simulink model "sus"  (Simulink 6.5)
settings: Solver=ode45  StartTime=0.0  StopTime=16  RelTol=1e-3
libraries: cdsFilt x266, cdsBitwise x92, cdsEpicsOut x84, cdsEpicsBinIn x56, cdsEpicsIn x20, cdsFiltCtrl x18, cdsMatrix x11, cdsSwitch x7, cdsWD x7, cdsFunctionCall x5, cdsRio1 x4, dac x3
(part 3 of 20)

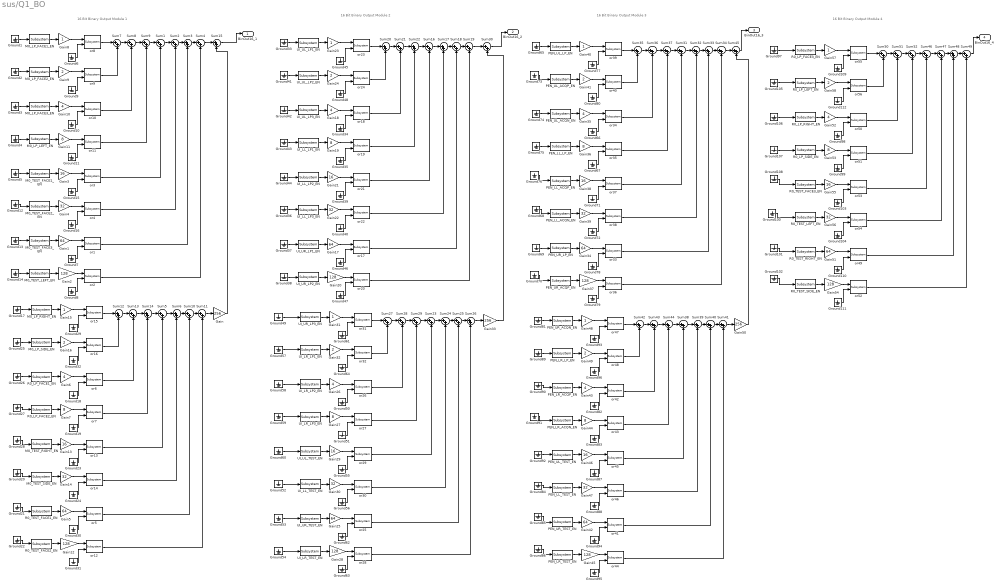
== system sus/Q1_BO ==
  note: 16 Bit Binary Output Module 1
  note: 16 Bit Binary Output Module 2
  note: 16 Bit Binary Output Module 3
  note: 16 Bit Binary Output Module 4
  Gain : Gain  Gain=256
  Gain{1,5,17,25,34,42,51} (7 alike) : Gain  Gain=64
  Gain{6,10,18,26,35,43,52} (7 alike) : Gain  Gain=4
  Gain{7,11,19,27,36,44,53} (7 alike) : Gain  Gain=8
  Gain{2,12,20,28,37,45,54} (7 alike) : Gain  Gain=128
  Gain{3,13,21,29,38,46,55} (7 alike) : Gain  Gain=16
  Gain{4,14,22,30,39,47,56} (7 alike) : Gain  Gain=32
  Gain{8,15,23,31,40,48,57} (7 alike) : Gain
  Gain{9,16,24,32,41,49,58} (7 alike) : Gain  Gain=2
  Gain33 : Gain  Gain=256
  Gain50 : Gain  Gain=256
  Ground{1..112} (112 alike) : Ground
  M0_LP_FACE1_EN : cdsEpicsBinIn/Subsystem  Tag=cdsEpicsBinIn  Description=|  SystemSampleTime=-1
      | Purpose:                                                                            
      | Create an EPICS binary (0 or 1) input channel to the FE realtime controls.          
      |                                                                                     
      | Operation:                                                                          
      | Outputs value from an EPICS ai record. Value is binary input (bi Epics record type).
      |                                                                                     
      | Usage:                                                                              
      | Name the part with the desired EPICS channel name.
      settings: AttributesFormatString=%<Tag>
  M0_LP_FACE2_EN : cdsEpicsBinIn/Subsystem  Tag=cdsEpicsBinIn  Description=|  SystemSampleTime=-1
      | Purpose:                                                                            
      | Create an EPICS binary (0 or 1) input channel to the FE realtime controls.          
      |                                                                                     
      | Operation:                                                                          
      | Outputs value from an EPICS ai record. Value is binary input (bi Epics record type).
      |                                                                                     
      | Usage:                                                                              
      | Name the part with the desired EPICS channel name.
      settings: AttributesFormatString=%<Tag>
  M0_LP_FACE3_EN : cdsEpicsBinIn/Subsystem  Tag=cdsEpicsBinIn  Description=|  SystemSampleTime=-1
      | Purpose:                                                                            
      | Create an EPICS binary (0 or 1) input channel to the FE realtime controls.          
      |                                                                                     
      | Operation:                                                                          
      | Outputs value from an EPICS ai record. Value is binary input (bi Epics record type).
      |                                                                                     
      | Usage:                                                                              
      | Name the part with the desired EPICS channel name.
      settings: AttributesFormatString=%<Tag>
  M0_LP_LEFT_EN : cdsEpicsBinIn/Subsystem  Tag=cdsEpicsBinIn  Description=|  SystemSampleTime=-1
      | Purpose:                                                                            
      | Create an EPICS binary (0 or 1) input channel to the FE realtime controls.          
      |                                                                                     
      | Operation:                                                                          
      | Outputs value from an EPICS ai record. Value is binary input (bi Epics record type).
      |                                                                                     
      | Usage:                                                                              
      | Name the part with the desired EPICS channel name.
      settings: AttributesFormatString=%<Tag>
  M0_LP_RIGHT_EN : cdsEpicsBinIn/Subsystem  Tag=cdsEpicsBinIn  Description=|  SystemSampleTime=-1
      | Purpose:                                                                            
      | Create an EPICS binary (0 or 1) input channel to the FE realtime controls.          
      |                                                                                     
      | Operation:                                                                          
      | Outputs value from an EPICS ai record. Value is binary input (bi Epics record type).
      |                                                                                     
      | Usage:                                                                              
      | Name the part with the desired EPICS channel name.
      settings: AttributesFormatString=%<Tag>
  M0_LP_SIDE_EN : cdsEpicsBinIn/Subsystem  Tag=cdsEpicsBinIn  Description=|  SystemSampleTime=-1
      | Purpose:                                                                            
      | Create an EPICS binary (0 or 1) input channel to the FE realtime controls.          
      |                                                                                     
      | Operation:                                                                          
      | Outputs value from an EPICS ai record. Value is binary input (bi Epics record type).
      |                                                                                     
      | Usage:                                                                              
      | Name the part with the desired EPICS channel name.
      settings: AttributesFormatString=%<Tag>
  M0_TEST_FACE1_EN : cdsEpicsBinIn/Subsystem  Tag=cdsEpicsBinIn  Description=|  SystemSampleTime=-1
      | Purpose:                                                                            
      | Create an EPICS binary (0 or 1) input channel to the FE realtime controls.          
      |                                                                                     
      | Operation:                                                                          
      | Outputs value from an EPICS ai record. Value is binary input (bi Epics record type).
      |                                                                                     
      | Usage:                                                                              
      | Name the part with the desired EPICS channel name.
      settings: AttributesFormatString=%<Tag>
  M0_TEST_FACE2_EN : cdsEpicsBinIn/Subsystem  Tag=cdsEpicsBinIn  Description=|  SystemSampleTime=-1
      | Purpose:                                                                            
      | Create an EPICS binary (0 or 1) input channel to the FE realtime controls.          
      |                                                                                     
      | Operation:                                                                          
      | Outputs value from an EPICS ai record. Value is binary input (bi Epics record type).
      |                                                                                     
      | Usage:                                                                              
      | Name the part with the desired EPICS channel name.
      settings: AttributesFormatString=%<Tag>
  M0_TEST_FACE3_EN : cdsEpicsBinIn/Subsystem  Tag=cdsEpicsBinIn  Description=|  SystemSampleTime=-1
      | Purpose:                                                                            
      | Create an EPICS binary (0 or 1) input channel to the FE realtime controls.          
      |                                                                                     
      | Operation:                                                                          
      | Outputs value from an EPICS ai record. Value is binary input (bi Epics record type).
      |                                                                                     
      | Usage:                                                                              
      | Name the part with the desired EPICS channel name.
      settings: AttributesFormatString=%<Tag>
  M0_TEST_LEFT_EN : cdsEpicsBinIn/Subsystem  Tag=cdsEpicsBinIn  Description=|  SystemSampleTime=-1
      | Purpose:                                                                            
      | Create an EPICS binary (0 or 1) input channel to the FE realtime controls.          
      |                                                                                     
      | Operation:                                                                          
      | Outputs value from an EPICS ai record. Value is binary input (bi Epics record type).
      |                                                                                     
      | Usage:                                                                              
      | Name the part with the desired EPICS channel name.
      settings: AttributesFormatString=%<Tag>
  M0_TEST_RIGHT_EN : cdsEpicsBinIn/Subsystem  Tag=cdsEpicsBinIn  Description=|  SystemSampleTime=-1
      | Purpose:                                                                            
      | Create an EPICS binary (0 or 1) input channel to the FE realtime controls.          
      |                                                                                     
      | Operation:                                                                          
      | Outputs value from an EPICS ai record. Value is binary input (bi Epics record type).
      |                                                                                     
      | Usage:                                                                              
      | Name the part with the desired EPICS channel name.
      settings: AttributesFormatString=%<Tag>
  M0_TEST_SIDE_EN : cdsEpicsBinIn/Subsystem  Tag=cdsEpicsBinIn  Description=|  SystemSampleTime=-1
      | Purpose:                                                                            
      | Create an EPICS binary (0 or 1) input channel to the FE realtime controls.          
      |                                                                                     
      | Operation:                                                                          
      | Outputs value from an EPICS ai record. Value is binary input (bi Epics record type).
      |                                                                                     
      | Usage:                                                                              
      | Name the part with the desired EPICS channel name.
      settings: AttributesFormatString=%<Tag>
  PEN_LL_ACQN_EN : cdsEpicsBinIn/Subsystem  Tag=cdsEpicsBinIn  Description=|  SystemSampleTime=-1
      | Purpose:                                                                            
      | Create an EPICS binary (0 or 1) input channel to the FE realtime controls.          
      |                                                                                     
      | Operation:                                                                          
      | Outputs value from an EPICS ai record. Value is binary input (bi Epics record type).
      |                                                                                     
      | Usage:                                                                              
      | Name the part with the desired EPICS channel name.
      settings: AttributesFormatString=%<Tag>
  PEN_LL_ACQP_EN : cdsEpicsBinIn/Subsystem  Tag=cdsEpicsBinIn  Description=|  SystemSampleTime=-1
      | Purpose:                                                                            
      | Create an EPICS binary (0 or 1) input channel to the FE realtime controls.          
      |                                                                                     
      | Operation:                                                                          
      | Outputs value from an EPICS ai record. Value is binary input (bi Epics record type).
      |                                                                                     
      | Usage:                                                                              
      | Name the part with the desired EPICS channel name.
      settings: AttributesFormatString=%<Tag>
  PEN_LL_LP_EN : cdsEpicsBinIn/Subsystem  Tag=cdsEpicsBinIn  Description=|  SystemSampleTime=-1
      | Purpose:                                                                            
      | Create an EPICS binary (0 or 1) input channel to the FE realtime controls.          
      |                                                                                     
      | Operation:                                                                          
      | Outputs value from an EPICS ai record. Value is binary input (bi Epics record type).
      |                                                                                     
      | Usage:                                                                              
      | Name the part with the desired EPICS channel name.
      settings: AttributesFormatString=%<Tag>
  PEN_LL_TEST_EN : cdsEpicsBinIn/Subsystem  Tag=cdsEpicsBinIn  Description=|  SystemSampleTime=-1
      | Purpose:                                                                            
      | Create an EPICS binary (0 or 1) input channel to the FE realtime controls.          
      |                                                                                     
      | Operation:                                                                          
      | Outputs value from an EPICS ai record. Value is binary input (bi Epics record type).
      |                                                                                     
      | Usage:                                                                              
      | Name the part with the desired EPICS channel name.
      settings: AttributesFormatString=%<Tag>
  PEN_LR_ACQN_EN : cdsEpicsBinIn/Subsystem  Tag=cdsEpicsBinIn  Description=|  SystemSampleTime=-1
      | Purpose:                                                                            
      | Create an EPICS binary (0 or 1) input channel to the FE realtime controls.          
      |                                                                                     
      | Operation:                                                                          
      | Outputs value from an EPICS ai record. Value is binary input (bi Epics record type).
      |                                                                                     
      | Usage:                                                                              
      | Name the part with the desired EPICS channel name.
      settings: AttributesFormatString=%<Tag>
  PEN_LR_ACQP_EN : cdsEpicsBinIn/Subsystem  Tag=cdsEpicsBinIn  Description=|  SystemSampleTime=-1
      | Purpose:                                                                            
      | Create an EPICS binary (0 or 1) input channel to the FE realtime controls.          
      |                                                                                     
      | Operation:                                                                          
      | Outputs value from an EPICS ai record. Value is binary input (bi Epics record type).
      |                                                                                     
      | Usage:                                                                              
      | Name the part with the desired EPICS channel name.
      settings: AttributesFormatString=%<Tag>
  PEN_LR_LP_EN : cdsEpicsBinIn/Subsystem  Tag=cdsEpicsBinIn  Description=|  SystemSampleTime=-1
      | Purpose:                                                                            
      | Create an EPICS binary (0 or 1) input channel to the FE realtime controls.          
      |                                                                                     
      | Operation:                                                                          
      | Outputs value from an EPICS ai record. Value is binary input (bi Epics record type).
      |                                                                                     
      | Usage:                                                                              
      | Name the part with the desired EPICS channel name.
      settings: AttributesFormatString=%<Tag>
  PEN_LR_TEST_EN : cdsEpicsBinIn/Subsystem  Tag=cdsEpicsBinIn  Description=|  SystemSampleTime=-1
      | Purpose:                                                                            
      | Create an EPICS binary (0 or 1) input channel to the FE realtime controls.          
      |                                                                                     
      | Operation:                                                                          
      | Outputs value from an EPICS ai record. Value is binary input (bi Epics record type).
      |                                                                                     
      | Usage:                                                                              
      | Name the part with the desired EPICS channel name.
      settings: AttributesFormatString=%<Tag>
  PEN_UL_ACQN_EN : cdsEpicsBinIn/Subsystem  Tag=cdsEpicsBinIn  Description=|  SystemSampleTime=-1
      | Purpose:                                                                            
      | Create an EPICS binary (0 or 1) input channel to the FE realtime controls.          
      |                                                                                     
      | Operation:                                                                          
      | Outputs value from an EPICS ai record. Value is binary input (bi Epics record type).
      |                                                                                     
      | Usage:                                                                              
      | Name the part with the desired EPICS channel name.
      settings: AttributesFormatString=%<Tag>
  PEN_UL_ACQP_EN : cdsEpicsBinIn/Subsystem  Tag=cdsEpicsBinIn  Description=|  SystemSampleTime=-1
      | Purpose:                                                                            
      | Create an EPICS binary (0 or 1) input channel to the FE realtime controls.          
      |                                                                                     
      | Operation:                                                                          
      | Outputs value from an EPICS ai record. Value is binary input (bi Epics record type).
      |                                                                                     
      | Usage:                                                                              
      | Name the part with the desired EPICS channel name.
      settings: AttributesFormatString=%<Tag>
  PEN_UL_LP_EN : cdsEpicsBinIn/Subsystem  Tag=cdsEpicsBinIn  Description=|  SystemSampleTime=-1
      | Purpose:                                                                            
      | Create an EPICS binary (0 or 1) input channel to the FE realtime controls.          
      |                                                                                     
      | Operation:                                                                          
      | Outputs value from an EPICS ai record. Value is binary input (bi Epics record type).
      |                                                                                     
      | Usage:                                                                              
      | Name the part with the desired EPICS channel name.
      settings: AttributesFormatString=%<Tag>
  PEN_UL_TEST_EN : cdsEpicsBinIn/Subsystem  Tag=cdsEpicsBinIn  Description=|  SystemSampleTime=-1
      | Purpose:                                                                            
      | Create an EPICS binary (0 or 1) input channel to the FE realtime controls.          
      |                                                                                     
      | Operation:                                                                          
      | Outputs value from an EPICS ai record. Value is binary input (bi Epics record type).
      |                                                                                     
      | Usage:                                                                              
      | Name the part with the desired EPICS channel name.
      settings: AttributesFormatString=%<Tag>
  PEN_UR_ACQN_EN : cdsEpicsBinIn/Subsystem  Tag=cdsEpicsBinIn  Description=|  SystemSampleTime=-1
      | Purpose:                                                                            
      | Create an EPICS binary (0 or 1) input channel to the FE realtime controls.          
      |                                                                                     
      | Operation:                                                                          
      | Outputs value from an EPICS ai record. Value is binary input (bi Epics record type).
      |                                                                                     
      | Usage:                                                                              
      | Name the part with the desired EPICS channel name.
      settings: AttributesFormatString=%<Tag>
  PEN_UR_ACQP_EN : cdsEpicsBinIn/Subsystem  Tag=cdsEpicsBinIn  Description=|  SystemSampleTime=-1
      | Purpose:                                                                            
      | Create an EPICS binary (0 or 1) input channel to the FE realtime controls.          
      |                                                                                     
      | Operation:                                                                          
      | Outputs value from an EPICS ai record. Value is binary input (bi Epics record type).
      |                                                                                     
      | Usage:                                                                              
      | Name the part with the desired EPICS channel name.
      settings: AttributesFormatString=%<Tag>
  PEN_UR_LP_EN : cdsEpicsBinIn/Subsystem  Tag=cdsEpicsBinIn  Description=|  SystemSampleTime=-1
      | Purpose:                                                                            
      | Create an EPICS binary (0 or 1) input channel to the FE realtime controls.          
      |                                                                                     
      | Operation:                                                                          
      | Outputs value from an EPICS ai record. Value is binary input (bi Epics record type).
      |                                                                                     
      | Usage:                                                                              
      | Name the part with the desired EPICS channel name.
      settings: AttributesFormatString=%<Tag>
  PEN_UR_TEST_EN : cdsEpicsBinIn/Subsystem  Tag=cdsEpicsBinIn  Description=|  SystemSampleTime=-1
      | Purpose:                                                                            
      | Create an EPICS binary (0 or 1) input channel to the FE realtime controls.          
      |                                                                                     
      | Operation:                                                                          
      | Outputs value from an EPICS ai record. Value is binary input (bi Epics record type).
      |                                                                                     
      | Usage:                                                                              
      | Name the part with the desired EPICS channel name.
      settings: AttributesFormatString=%<Tag>
  R0_LP_FACE1_EN : cdsEpicsBinIn/Subsystem  Tag=cdsEpicsBinIn  Description=|  SystemSampleTime=-1
      | Purpose:                                                                            
      | Create an EPICS binary (0 or 1) input channel to the FE realtime controls.          
      |                                                                                     
      | Operation:                                                                          
      | Outputs value from an EPICS ai record. Value is binary input (bi Epics record type).
      |                                                                                     
      | Usage:                                                                              
      | Name the part with the desired EPICS channel name.
      settings: AttributesFormatString=%<Tag>
  R0_LP_FACE2_EN : cdsEpicsBinIn/Subsystem  Tag=cdsEpicsBinIn  Description=|  SystemSampleTime=-1
      | Purpose:                                                                            
      | Create an EPICS binary (0 or 1) input channel to the FE realtime controls.          
      |                                                                                     
      | Operation:                                                                          
      | Outputs value from an EPICS ai record. Value is binary input (bi Epics record type).
      |                                                                                     
      | Usage:                                                                              
      | Name the part with the desired EPICS channel name.
      settings: AttributesFormatString=%<Tag>
  R0_LP_FACE3_EN : cdsEpicsBinIn/Subsystem  Tag=cdsEpicsBinIn  Description=|  SystemSampleTime=-1
      | Purpose:                                                                            
      | Create an EPICS binary (0 or 1) input channel to the FE realtime controls.          
      |                                                                                     
      | Operation:                                                                          
      | Outputs value from an EPICS ai record. Value is binary input (bi Epics record type).
      |                                                                                     
      | Usage:                                                                              
      | Name the part with the desired EPICS channel name.
      settings: AttributesFormatString=%<Tag>
  R0_LP_LEFT_EN : cdsEpicsBinIn/Subsystem  Tag=cdsEpicsBinIn  Description=|  SystemSampleTime=-1
      | Purpose:                                                                            
      | Create an EPICS binary (0 or 1) input channel to the FE realtime controls.          
      |                                                                                     
      | Operation:                                                                          
      | Outputs value from an EPICS ai record. Value is binary input (bi Epics record type).
      |                                                                                     
      | Usage:                                                                              
      | Name the part with the desired EPICS channel name.
      settings: AttributesFormatString=%<Tag>
  R0_LP_RIGHT_EN : cdsEpicsBinIn/Subsystem  Tag=cdsEpicsBinIn  Description=|  SystemSampleTime=-1
      | Purpose:                                                                            
      | Create an EPICS binary (0 or 1) input channel to the FE realtime controls.          
      |                                                                                     
      | Operation:                                                                          
      | Outputs value from an EPICS ai record. Value is binary input (bi Epics record type).
      |                                                                                     
      | Usage:                                                                              
      | Name the part with the desired EPICS channel name.
      settings: AttributesFormatString=%<Tag>
  R0_LP_SIDE_EN : cdsEpicsBinIn/Subsystem  Tag=cdsEpicsBinIn  Description=|  SystemSampleTime=-1
      | Purpose:                                                                            
      | Create an EPICS binary (0 or 1) input channel to the FE realtime controls.          
      |                                                                                     
      | Operation:                                                                          
      | Outputs value from an EPICS ai record. Value is binary input (bi Epics record type).
      |                                                                                     
      | Usage:                                                                              
      | Name the part with the desired EPICS channel name.
      settings: AttributesFormatString=%<Tag>
  R0_TEST_FACE1_EN : cdsEpicsBinIn/Subsystem  Tag=cdsEpicsBinIn  Description=|  SystemSampleTime=-1
      | Purpose:                                                                            
      | Create an EPICS binary (0 or 1) input channel to the FE realtime controls.          
      |                                                                                     
      | Operation:                                                                          
      | Outputs value from an EPICS ai record. Value is binary input (bi Epics record type).
      |                                                                                     
      | Usage:                                                                              
      | Name the part with the desired EPICS channel name.
      settings: AttributesFormatString=%<Tag>
  R0_TEST_FACE2_EN : cdsEpicsBinIn/Subsystem  Tag=cdsEpicsBinIn  Description=|  SystemSampleTime=-1
      | Purpose:                                                                            
      | Create an EPICS binary (0 or 1) input channel to the FE realtime controls.          
      |                                                                                     
      | Operation:                                                                          
      | Outputs value from an EPICS ai record. Value is binary input (bi Epics record type).
      |                                                                                     
      | Usage:                                                                              
      | Name the part with the desired EPICS channel name.
      settings: AttributesFormatString=%<Tag>
  R0_TEST_FACE3_EN : cdsEpicsBinIn/Subsystem  Tag=cdsEpicsBinIn  Description=|  SystemSampleTime=-1
      | Purpose:                                                                            
      | Create an EPICS binary (0 or 1) input channel to the FE realtime controls.          
      |                                                                                     
      | Operation:                                                                          
      | Outputs value from an EPICS ai record. Value is binary input (bi Epics record type).
      |                                                                                     
      | Usage:                                                                              
      | Name the part with the desired EPICS channel name.
      settings: AttributesFormatString=%<Tag>
  R0_TEST_LEFT_EN : cdsEpicsBinIn/Subsystem  Tag=cdsEpicsBinIn  Description=|  SystemSampleTime=-1
      | Purpose:                                                                            
      | Create an EPICS binary (0 or 1) input channel to the FE realtime controls.          
      |                                                                                     
      | Operation:                                                                          
      | Outputs value from an EPICS ai record. Value is binary input (bi Epics record type).
      |                                                                                     
      | Usage:                                                                              
      | Name the part with the desired EPICS channel name.
      settings: AttributesFormatString=%<Tag>
  R0_TEST_RIGHT_EN : cdsEpicsBinIn/Subsystem  Tag=cdsEpicsBinIn  Description=|  SystemSampleTime=-1
      | Purpose:                                                                            
      | Create an EPICS binary (0 or 1) input channel to the FE realtime controls.          
      |                                                                                     
      | Operation:                                                                          
      | Outputs value from an EPICS ai record. Value is binary input (bi Epics record type).
      |                                                                                     
      | Usage:                                                                              
      | Name the part with the desired EPICS channel name.
      settings: AttributesFormatString=%<Tag>
  R0_TEST_SIDE_EN : cdsEpicsBinIn/Subsystem  Tag=cdsEpicsBinIn  Description=|  SystemSampleTime=-1
      | Purpose:                                                                            
      | Create an EPICS binary (0 or 1) input channel to the FE realtime controls.          
      |                                                                                     
      | Operation:                                                                          
      | Outputs value from an EPICS ai record. Value is binary input (bi Epics record type).
      |                                                                                     
      | Usage:                                                                              
      | Name the part with the desired EPICS channel name.
      settings: AttributesFormatString=%<Tag>
  Sum{1..52} (52 alike) : Sum  Inputs=|++
  UI_LL_LP1_EN : cdsEpicsBinIn/Subsystem  Tag=cdsEpicsBinIn  Description=|  SystemSampleTime=-1
      | Purpose:                                                                            
      | Create an EPICS binary (0 or 1) input channel to the FE realtime controls.          
      |                                                                                     
      | Operation:                                                                          
      | Outputs value from an EPICS ai record. Value is binary input (bi Epics record type).
      |                                                                                     
      | Usage:                                                                              
      | Name the part with the desired EPICS channel name.
      settings: AttributesFormatString=%<Tag>
  UI_LL_LP2_EN : cdsEpicsBinIn/Subsystem  Tag=cdsEpicsBinIn  Description=|  SystemSampleTime=-1
      | Purpose:                                                                            
      | Create an EPICS binary (0 or 1) input channel to the FE realtime controls.          
      |                                                                                     
      | Operation:                                                                          
      | Outputs value from an EPICS ai record. Value is binary input (bi Epics record type).
      |                                                                                     
      | Usage:                                                                              
      | Name the part with the desired EPICS channel name.
      settings: AttributesFormatString=%<Tag>
  UI_LL_LP3_EN : cdsEpicsBinIn/Subsystem  Tag=cdsEpicsBinIn  Description=|  SystemSampleTime=-1
      | Purpose:                                                                            
      | Create an EPICS binary (0 or 1) input channel to the FE realtime controls.          
      |                                                                                     
      | Operation:                                                                          
      | Outputs value from an EPICS ai record. Value is binary input (bi Epics record type).
      |                                                                                     
      | Usage:                                                                              
      | Name the part with the desired EPICS channel name.
      settings: AttributesFormatString=%<Tag>
  UI_LL_TEST_EN : cdsEpicsBinIn/Subsystem  Tag=cdsEpicsBinIn  Description=|  SystemSampleTime=-1
      | Purpose:                                                                            
      | Create an EPICS binary (0 or 1) input channel to the FE realtime controls.          
      |                                                                                     
      | Operation:                                                                          
      | Outputs value from an EPICS ai record. Value is binary input (bi Epics record type).
      |                                                                                     
      | Usage:                                                                              
      | Name the part with the desired EPICS channel name.
      settings: AttributesFormatString=%<Tag>
  UI_LR_LP1_EN : cdsEpicsBinIn/Subsystem  Tag=cdsEpicsBinIn  Description=|  SystemSampleTime=-1
      | Purpose:                                                                            
      | Create an EPICS binary (0 or 1) input channel to the FE realtime controls.          
      |                                                                                     
      | Operation:                                                                          
      | Outputs value from an EPICS ai record. Value is binary input (bi Epics record type).
      |                                                                                     
      | Usage:                                                                              
      | Name the part with the desired EPICS channel name.
      settings: AttributesFormatString=%<Tag>
  UI_LR_LP2_EN : cdsEpicsBinIn/Subsystem  Tag=cdsEpicsBinIn  Description=|  SystemSampleTime=-1
      | Purpose:                                                                            
      | Create an EPICS binary (0 or 1) input channel to the FE realtime controls.          
      |                                                                                     
      | Operation:                                                                          
      | Outputs value from an EPICS ai record. Value is binary input (bi Epics record type).
      |                                                                                     
      | Usage:                                                                              
      | Name the part with the desired EPICS channel name.
      settings: AttributesFormatString=%<Tag>
  UI_LR_LP3_EN : cdsEpicsBinIn/Subsystem  Tag=cdsEpicsBinIn  Description=|  SystemSampleTime=-1
      | Purpose:                                                                            
      | Create an EPICS binary (0 or 1) input channel to the FE realtime controls.          
      |                                                                                     
      | Operation:                                                                          
      | Outputs value from an EPICS ai record. Value is binary input (bi Epics record type).
      |                                                                                     
      | Usage:                                                                              
      | Name the part with the desired EPICS channel name.
      settings: AttributesFormatString=%<Tag>
  UI_LR_TEST_EN : cdsEpicsBinIn/Subsystem  Tag=cdsEpicsBinIn  Description=|  SystemSampleTime=-1
      | Purpose:                                                                            
      | Create an EPICS binary (0 or 1) input channel to the FE realtime controls.          
      |                                                                                     
      | Operation:                                                                          
      | Outputs value from an EPICS ai record. Value is binary input (bi Epics record type).
      |                                                                                     
      | Usage:                                                                              
      | Name the part with the desired EPICS channel name.
      settings: AttributesFormatString=%<Tag>
  UI_UL_LP1_EN : cdsEpicsBinIn/Subsystem  Tag=cdsEpicsBinIn  Description=|  SystemSampleTime=-1
      | Purpose:                                                                            
      | Create an EPICS binary (0 or 1) input channel to the FE realtime controls.          
      |                                                                                     
      | Operation:                                                                          
      | Outputs value from an EPICS ai record. Value is binary input (bi Epics record type).
      |                                                                                     
      | Usage:                                                                              
      | Name the part with the desired EPICS channel name.
      settings: AttributesFormatString=%<Tag>
  UI_UL_LP2_EN : cdsEpicsBinIn/Subsystem  Tag=cdsEpicsBinIn  Description=|  SystemSampleTime=-1
      | Purpose:                                                                            
      | Create an EPICS binary (0 or 1) input channel to the FE realtime controls.          
      |                                                                                     
      | Operation:                                                                          
      | Outputs value from an EPICS ai record. Value is binary input (bi Epics record type).
      |                                                                                     
      | Usage:                                                                              
      | Name the part with the desired EPICS channel name.
      settings: AttributesFormatString=%<Tag>
  UI_UL_LP3_EN : cdsEpicsBinIn/Subsystem  Tag=cdsEpicsBinIn  Description=|  SystemSampleTime=-1
      | Purpose:                                                                            
      | Create an EPICS binary (0 or 1) input channel to the FE realtime controls.          
      |                                                                                     
      | Operation:                                                                          
      | Outputs value from an EPICS ai record. Value is binary input (bi Epics record type).
      |                                                                                     
      | Usage:                                                                              
      | Name the part with the desired EPICS channel name.
      settings: AttributesFormatString=%<Tag>
  UI_UL_TEST_EN : cdsEpicsBinIn/Subsystem  Tag=cdsEpicsBinIn  Description=|  SystemSampleTime=-1
      | Purpose:                                                                            
      | Create an EPICS binary (0 or 1) input channel to the FE realtime controls.          
      |                                                                                     
      | Operation:                                                                          
      | Outputs value from an EPICS ai record. Value is binary input (bi Epics record type).
      |                                                                                     
      | Usage:                                                                              
      | Name the part with the desired EPICS channel name.
      settings: AttributesFormatString=%<Tag>
  UI_UR_LP1_EN : cdsEpicsBinIn/Subsystem  Tag=cdsEpicsBinIn  Description=|  SystemSampleTime=-1
      | Purpose:                                                                            
      | Create an EPICS binary (0 or 1) input channel to the FE realtime controls.          
      |                                                                                     
      | Operation:                                                                          
      | Outputs value from an EPICS ai record. Value is binary input (bi Epics record type).
      |                                                                                     
      | Usage:                                                                              
      | Name the part with the desired EPICS channel name.
      settings: AttributesFormatString=%<Tag>
  UI_UR_LP2_EN : cdsEpicsBinIn/Subsystem  Tag=cdsEpicsBinIn  Description=|  SystemSampleTime=-1
      | Purpose:                                                                            
      | Create an EPICS binary (0 or 1) input channel to the FE realtime controls.          
      |                                                                                     
      | Operation:                                                                          
      | Outputs value from an EPICS ai record. Value is binary input (bi Epics record type).
      |                                                                                     
      | Usage:                                                                              
      | Name the part with the desired EPICS channel name.
      settings: AttributesFormatString=%<Tag>
  UI_UR_LP3_EN : cdsEpicsBinIn/Subsystem  Tag=cdsEpicsBinIn  Description=|  SystemSampleTime=-1
      | Purpose:                                                                            
      | Create an EPICS binary (0 or 1) input channel to the FE realtime controls.          
      |                                                                                     
      | Operation:                                                                          
      | Outputs value from an EPICS ai record. Value is binary input (bi Epics record type).
      |                                                                                     
      | Usage:                                                                              
      | Name the part with the desired EPICS channel name.
      settings: AttributesFormatString=%<Tag>
  UI_UR_TEST_EN : cdsEpicsBinIn/Subsystem  Tag=cdsEpicsBinIn  Description=|  SystemSampleTime=-1
      | Purpose:                                                                            
      | Create an EPICS binary (0 or 1) input channel to the FE realtime controls.          
      |                                                                                     
      | Operation:                                                                          
      | Outputs value from an EPICS ai record. Value is binary input (bi Epics record type).
      |                                                                                     
      | Usage:                                                                              
      | Name the part with the desired EPICS channel name.
      settings: AttributesFormatString=%<Tag>
  or{1..56} (56 alike) : cdsBitwise/Subsystem  Tag=cdsBitwise  SystemSampleTime=-1
      settings: AttributesFormatString=%<Tag>
  BinOut16_1 : Outport
  BinOut16_2 : Outport  Port=2
  BinOut16_3 : Outport  Port=3
  BinOut16_4 : Outport  Port=4
  wires:
  Sum15/1 -> BinOut16_1/1
  Gain/1 -> Sum15/2
  or12/1 -> Sum11/2
  or5/1 -> Sum10/2
  or14/1 -> Sum6/2
  or13/1 -> Sum5/2
  Sum11/1 -> Gain/1
  Sum10/1 -> Sum11/1
  Sum6/1 -> Sum10/1
  Sum5/1 -> Sum6/1
  Sum14/1 -> Sum5/1
  Ground20/1 -> M0_TEST_SIDE_EN/1
  Ground21/1 -> R0_TEST_FACE1_EN/1
  Ground22/1 -> R0_TEST_FACE2_EN/1
  Ground28/1 -> M0_TEST_RIGHT_EN/1
  Ground31/1 -> or12/2
  R0_TEST_FACE2_EN/1 -> Gain12/1
  Gain12/1 -> or12/1
  Ground30/1 -> or5/2
  R0_TEST_FACE1_EN/1 -> Gain5/1
  Gain5/1 -> or5/1
  Ground23/1 -> or13/2
  M0_TEST_RIGHT_EN/1 -> Gain13/1
  Gain13/1 -> or13/1
  Ground24/1 -> or14/2
  M0_TEST_SIDE_EN/1 -> Gain14/1
  Gain14/1 -> or14/1
  Ground25/1 -> M0_LP_SIDE_EN/1
  Ground26/1 -> R0_LP_FACE1_EN/1
  Ground27/1 -> R0_LP_FACE2_EN/1
  Ground17/1 -> M0_LP_RIGHT_EN/1
  or7/1 -> Sum14/2
  Sum13/1 -> Sum14/1
  Ground19/1 -> or7/2
  R0_LP_FACE2_EN/1 -> Gain7/1
  Gain7/1 -> or7/1
  or6/1 -> Sum13/2
  Sum12/1 -> Sum13/1
  Ground18/1 -> or6/2
  R0_LP_FACE1_EN/1 -> Gain6/1
  Gain6/1 -> or6/1
  Ground29/1 -> or15/2
  M0_LP_RIGHT_EN/1 -> Gain15/1
  Gain15/1 -> or15/1
  or15/1 -> Sum12/1
  Ground32/1 -> or16/2
  M0_LP_SIDE_EN/1 -> Gain16/1
  Gain16/1 -> or16/1
  or16/1 -> Sum12/2
  or2/1 -> Sum4/2
  or1/1 -> Sum3/2
  or4/1 -> Sum2/2
  or3/1 -> Sum1/2
  Sum4/1 -> Sum15/1
  Sum3/1 -> Sum4/1
  Sum2/1 -> Sum3/1
  Sum1/1 -> Sum2/1
  Sum9/1 -> Sum1/1
  Ground12/1 -> M0_TEST_FACE2_EN/1
  Ground13/1 -> M0_TEST_FACE3_EN/1
  Ground14/1 -> M0_TEST_LEFT_EN/1
  Ground5/1 -> M0_TEST_FACE1_EN/1
  Ground8/1 -> or2/2
  M0_TEST_LEFT_EN/1 -> Gain2/1
  Gain2/1 -> or2/1
  Ground7/1 -> or1/2
  M0_TEST_FACE3_EN/1 -> Gain1/1
  Gain1/1 -> or1/1
  Ground15/1 -> or3/2
  M0_TEST_FACE1_EN/1 -> Gain3/1
  Gain3/1 -> or3/1
  Ground16/1 -> or4/2
  M0_TEST_FACE2_EN/1 -> Gain4/1
  Gain4/1 -> or4/1
  Ground2/1 -> M0_LP_FACE2_EN/1
  Ground3/1 -> M0_LP_FACE3_EN/1
  Ground4/1 -> M0_LP_LEFT_EN/1
  Ground1/1 -> M0_LP_FACE1_EN/1
  or11/1 -> Sum9/2
  Sum8/1 -> Sum9/1
  Ground11/1 -> or11/2
  M0_LP_LEFT_EN/1 -> Gain11/1
  Gain11/1 -> or11/1
  or10/1 -> Sum8/2
  Sum7/1 -> Sum8/1
  Ground10/1 -> or10/2
  M0_LP_FACE3_EN/1 -> Gain10/1
  Gain10/1 -> or10/1
  Ground6/1 -> or8/2
  M0_LP_FACE1_EN/1 -> Gain8/1
  Gain8/1 -> or8/1
  or8/1 -> Sum7/1
  Ground9/1 -> or9/2
  M0_LP_FACE2_EN/1 -> Gain9/1
  Gain9/1 -> or9/1
  or9/1 -> Sum7/2
  or24/1 -> Sum20/2
  Gain24/1 -> or24/1
  UI_UL_LP2_EN/1 -> Gain24/1
  Ground48/1 -> or24/2
  or23/1 -> Sum20/1
  Gain23/1 -> or23/1
  UI_UL_LP1_EN/1 -> Gain23/1
  Ground45/1 -> or23/2
  Gain18/1 -> or18/1
  UI_UL_LP3_EN/1 -> Gain18/1
  Ground34/1 -> or18/2
  Sum20/1 -> Sum21/1
  or18/1 -> Sum21/2
  Gain19/1 -> or19/1
  UI_LL_LP1_EN/1 -> Gain19/1
  Ground35/1 -> or19/2
  Sum21/1 -> Sum22/1
  or19/1 -> Sum22/2
  Ground33/1 -> UI_UL_LP1_EN/1
  Ground43/1 -> UI_LL_LP1_EN/1
  Ground42/1 -> UI_UL_LP3_EN/1
  Ground41/1 -> UI_UL_LP2_EN/1
  Gain22/1 -> or22/1
  UI_LL_LP3_EN/1 -> Gain22/1
  Ground40/1 -> or22/2
  Gain21/1 -> or21/1
  UI_LL_LP2_EN/1 -> Gain21/1
  Ground39/1 -> or21/2
  Gain17/1 -> or17/1
  UI_UR_LP1_EN/1 -> Gain17/1
  Ground46/1 -> or17/2
  Gain20/1 -> or20/1
  UI_UR_LP2_EN/1 -> Gain20/1
  Ground47/1 -> or20/2
  Ground44/1 -> UI_LL_LP2_EN/1
  Ground38/1 -> UI_UR_LP2_EN/1
  Ground37/1 -> UI_UR_LP1_EN/1
  Ground36/1 -> UI_LL_LP3_EN/1
  Sum22/1 -> Sum16/1
  Sum16/1 -> Sum17/1
  Sum17/1 -> Sum18/1
  Sum18/1 -> Sum19/1
  Sum19/1 -> Sum30/1
  or21/1 -> Sum16/2
  or22/1 -> Sum17/2
  or17/1 -> Sum18/2
  or20/1 -> Sum19/2
  or32/1 -> Sum27/2
  Gain32/1 -> or32/1
  UI_LR_LP1_EN/1 -> Gain32/1
  Ground64/1 -> or32/2
  or31/1 -> Sum27/1
  Gain31/1 -> or31/1
  UI_UR_LP3_EN/1 -> Gain31/1
  Ground61/1 -> or31/2
  Gain26/1 -> or26/1
  UI_LR_LP2_EN/1 -> Gain26/1
  Ground50/1 -> or26/2
  Sum27/1 -> Sum28/1
  or26/1 -> Sum28/2
  Gain27/1 -> or27/1
  UI_LR_LP3_EN/1 -> Gain27/1
  Ground51/1 -> or27/2
  Sum28/1 -> Sum29/1
  or27/1 -> Sum29/2
  Ground49/1 -> UI_UR_LP3_EN/1
  Ground59/1 -> UI_LR_LP3_EN/1
  Ground58/1 -> UI_LR_LP2_EN/1
  Ground57/1 -> UI_LR_LP1_EN/1
  Gain30/1 -> or30/1
  UI_LL_TEST_EN/1 -> Gain30/1
  Ground56/1 -> or30/2
  Gain29/1 -> or29/1
  UI_UL_TEST_EN/1 -> Gain29/1
  Ground55/1 -> or29/2
  Gain25/1 -> or25/1
  UI_UR_TEST_EN/1 -> Gain25/1
  Ground62/1 -> or25/2
  Gain28/1 -> or28/1
  UI_LR_TEST_EN/1 -> Gain28/1
  Ground63/1 -> or28/2
  Ground60/1 -> UI_UL_TEST_EN/1
  Ground54/1 -> UI_LR_TEST_EN/1
  Ground53/1 -> UI_UR_TEST_EN/1
  Ground52/1 -> UI_LL_TEST_EN/1
  Sum29/1 -> Sum23/1
  Sum23/1 -> Sum24/1
  Sum24/1 -> Sum25/1
  Sum25/1 -> Sum26/1
  Sum26/1 -> Gain33/1
  or29/1 -> Sum23/2
  or30/1 -> Sum24/2
  or25/1 -> Sum25/2
  or28/1 -> Sum26/2
  Gain33/1 -> Sum30/2
  Sum30/1 -> BinOut16_2/1
  or40/1 -> Sum35/2
  Gain41/1 -> or40/1
  PEN_UL_ACQP_EN/1 -> Gain41/1
  Ground80/1 -> or40/2
  or39/1 -> Sum35/1
  Gain40/1 -> or39/1
  PEN_UL_LP_EN/1 -> Gain40/1
  Ground77/1 -> or39/2
  Gain35/1 -> or34/1
  PEN_UL_ACQN_EN/1 -> Gain35/1
  Ground66/1 -> or34/2
  Sum35/1 -> Sum36/1
  or34/1 -> Sum36/2
  Gain36/1 -> or35/1
  PEN_LL_LP_EN/1 -> Gain36/1
  Ground67/1 -> or35/2
  Sum36/1 -> Sum37/1
  or35/1 -> Sum37/2
  Ground65/1 -> PEN_UL_LP_EN/1
  Ground75/1 -> PEN_LL_LP_EN/1
  Ground74/1 -> PEN_UL_ACQN_EN/1
  Ground73/1 -> PEN_UL_ACQP_EN/1
  Gain39/1 -> or38/1
  PEN_LL_ACQN_EN/1 -> Gain39/1
  Ground72/1 -> or38/2
  Gain38/1 -> or37/1
  PEN_LL_ACQP_EN/1 -> Gain38/1
  Ground71/1 -> or37/2
  Gain34/1 -> or33/1
  PEN_UR_LP_EN/1 -> Gain34/1
  Ground78/1 -> or33/2
  Gain37/1 -> or36/1
  PEN_UR_ACQP_EN/1 -> Gain37/1
  Ground79/1 -> or36/2
  Ground76/1 -> PEN_LL_ACQP_EN/1
  Ground70/1 -> PEN_UR_ACQP_EN/1
  Ground69/1 -> PEN_UR_LP_EN/1
  Ground68/1 -> PEN_LL_ACQN_EN/1
  Sum37/1 -> Sum31/1
  Sum31/1 -> Sum32/1
  Sum32/1 -> Sum33/1
  Sum33/1 -> Sum34/1
  Sum34/1 -> Sum45/1
  or37/1 -> Sum31/2
  or38/1 -> Sum32/2
  or33/1 -> Sum33/2
  or36/1 -> Sum34/2
  or48/1 -> Sum42/2
  Gain49/1 -> or48/1
  PEN_LR_LP_EN/1 -> Gain49/1
  Ground96/1 -> or48/2
  or47/1 -> Sum42/1
  Gain48/1 -> or47/1
  PEN_UR_ACQN_EN/1 -> Gain48/1
  Ground93/1 -> or47/2
  Gain43/1 -> or42/1
  PEN_LR_ACQP_EN/1 -> Gain43/1
  Ground82/1 -> or42/2
  Sum42/1 -> Sum43/1
  or42/1 -> Sum43/2
  Gain44/1 -> or43/1
  PEN_LR_ACQN_EN/1 -> Gain44/1
  Ground83/1 -> or43/2
  Sum43/1 -> Sum44/1
  or43/1 -> Sum44/2
  Ground81/1 -> PEN_UR_ACQN_EN/1
  Ground91/1 -> PEN_LR_ACQN_EN/1
  Ground90/1 -> PEN_LR_ACQP_EN/1
  Ground89/1 -> PEN_LR_LP_EN/1
  Gain47/1 -> or46/1
  PEN_LL_TEST_EN/1 -> Gain47/1
  Ground88/1 -> or46/2
  Gain46/1 -> or45/1
  PEN_UL_TEST_EN/1 -> Gain46/1
  Ground87/1 -> or45/2
  Gain42/1 -> or41/1
  PEN_UR_TEST_EN/1 -> Gain42/1
  Ground94/1 -> or41/2
  Gain45/1 -> or44/1
  PEN_LR_TEST_EN/1 -> Gain45/1
  Ground95/1 -> or44/2
  Ground92/1 -> PEN_UL_TEST_EN/1
  Ground86/1 -> PEN_LR_TEST_EN/1
  Ground85/1 -> PEN_UR_TEST_EN/1
  Ground84/1 -> PEN_LL_TEST_EN/1
  Sum44/1 -> Sum38/1
  Sum38/1 -> Sum39/1
  Sum39/1 -> Sum40/1
  Sum40/1 -> Sum41/1
  Sum41/1 -> Gain50/1
  or45/1 -> Sum38/2
  or46/1 -> Sum39/2
  or41/1 -> Sum40/2
  or44/1 -> Sum41/2
  Gain50/1 -> Sum45/2
  Sum45/1 -> BinOut16_3/1
  or56/1 -> Sum50/2
  Gain58/1 -> or56/1
  R0_LP_LEFT_EN/1 -> Gain58/1
  Ground112/1 -> or56/2
  or55/1 -> Sum50/1
  Gain57/1 -> or55/1
  R0_LP_FACE3_EN/1 -> Gain57/1
  Ground109/1 -> or55/2
  Gain52/1 -> or50/1
  R0_LP_RIGHT_EN/1 -> Gain52/1
  Ground98/1 -> or50/2
  Sum50/1 -> Sum51/1
  or50/1 -> Sum51/2
  Gain53/1 -> or51/1
  R0_LP_SIDE_EN/1 -> Gain53/1
  Ground99/1 -> or51/2
  Sum51/1 -> Sum52/1
  or51/1 -> Sum52/2
  Ground97/1 -> R0_LP_FACE3_EN/1
  Ground107/1 -> R0_LP_SIDE_EN/1
  Ground106/1 -> R0_LP_RIGHT_EN/1
  Ground105/1 -> R0_LP_LEFT_EN/1
  Gain56/1 -> or54/1
  R0_TEST_LEFT_EN/1 -> Gain56/1
  Ground104/1 -> or54/2
  Gain55/1 -> or53/1
  R0_TEST_FACE3_EN/1 -> Gain55/1
  Ground103/1 -> or53/2
  Gain51/1 -> or49/1
  R0_TEST_RIGHT_EN/1 -> Gain51/1
  Ground110/1 -> or49/2
  Gain54/1 -> or52/1
  R0_TEST_SIDE_EN/1 -> Gain54/1
  Ground111/1 -> or52/2
  Ground108/1 -> R0_TEST_FACE3_EN/1
  Ground102/1 -> R0_TEST_SIDE_EN/1
  Ground101/1 -> R0_TEST_RIGHT_EN/1
  Ground100/1 -> R0_TEST_LEFT_EN/1
  Sum52/1 -> Sum46/1
  Sum46/1 -> Sum47/1
  Sum47/1 -> Sum48/1
  Sum48/1 -> Sum49/1
  Sum49/1 -> BinOut16_4/1
  or53/1 -> Sum46/2
  or54/1 -> Sum47/2
  or49/1 -> Sum48/2
  or52/1 -> Sum49/2
